simulink model "stateflow_AndOrDecomposition"  (R2015b)
settings: Solver=ode45  StartTime=0.0  StopTime=10.0  RelTol=1e-3
settings Model: Creator=ladmin  LastModifiedBy=ladmin
settings DataIOCC: SaveFormat=Array
settings DebuggingCC: SolverPrmCheckMsg=warning
settings GRTTargetCC: GeneratePreprocessorConditionals=Disable all
settings ConfigComp: CovModelRefEnable=Off  CovSFcnEnable=off

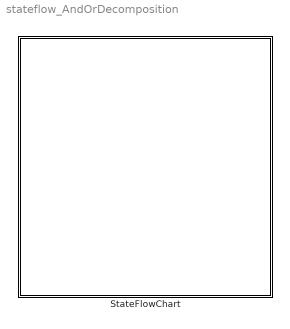
== system stateflow_AndOrDecomposition ==
  StateFlowChart : Stateflow chart  TreatAsAtomicUnit=on

== stateflow chart stateflow_AndOrDecomposition/StateFlowChart ==
  state OrState
    state SubState1InOr
    state SubState2InOr
  state AndState
    state SubState2InAnd [parallel]
      settings: executionOrder=1
    state SubState1InAnd [parallel]
      settings: executionOrder=2
